simulink model "VehDymcModel_Outputer"  (R2022b)
settings: Solver=ode4  StartTime=0.0  StopTime=DrvCycLen  RelTol=1e-3
model workspace (MAT data in the model file):
  socvcb = containers.Map
  socvcb.serialization.keys = {}
  socvcb.serialization.values = {}
  socvcb.serialization.uniformity = 0
  socvcb.serialization.keyType = 'double'
  socvcb.serialization.valueType = 'any'
values from neighbouring files (symbols this model uses):
  DCAC_eff = 0.95    [FCEV_original_data.mat]
  m = Time_sample    [Config_c22100601.m]    (also in Config_c22100701.m)
  MC_eff_brk_average = 0.810578512397    [FCEV_original_data.mat]
  MC_eff_dri_average = 0.810578512397    [FCEV_original_data.mat]
  MC_inertia = 0.06    [FCEV_original_data.mat]
  MC_ori_eff = [0.7 0.78 0.85 0.86 0.81 0.82 0.79 0.78 0.78 0.78 0.78 0.7 ... (231 elements, 11x21)]    [FCEV_original_data.mat]
  MC_ori_power_brk_req_kW = [0 -28.3912930389 -56.7825860779 -85.1738791168 -113.565172156 -141.956465195 -170.347758234 -198.739051273 -227.130344311 -255.52163735 -283.912930389 0 ... (121 elements, 11x11)]    [FCEV_original_data.mat]
  MC_ori_power_dri_req_kW = [0 0 0 0 0 0 0 0 0 0 0 0 ... (121 elements, 11x11)]    [FCEV_original_data.mat]
  MC_ori_spd_rpm = [0 1000 2000 3000 4000 5000 6000 7000 8000 9000 10000]    [FCEV_original_data.mat]
  MC_ori_trq_brk_max_Nm = [-271.1368 -271.1368 -271.1368 -237.5159 -178.1369 -142.4824 -118.7579 -101.8119 -89.0685 -79.172 -71.1734]    [FCEV_original_data.mat]
  MC_ori_trq_brk_Nm = [-271.136848522 -244.02316367 -216.909478817 -189.795793965 -162.682109113 -135.568424261 -108.454739409 -81.3410545565 -54.2273697044 -27.1136848522 0]    [FCEV_original_data.mat]
  MC_ori_trq_dri_max_Nm = [271.1368 271.1368 271.1368 237.5159 178.1369 142.4824 118.7579 101.8119 89.0685 79.172 71.1734]    [FCEV_original_data.mat]
  MC_ori_trq_dri_Nm = [0 27.1136848522 54.2273697044 81.3410545565 108.454739409 135.568424261 162.682109113 189.795793965 216.909478817 244.02316367 271.136848522]    [FCEV_original_data.mat]
  MC_ori_trq_Nm = [-271.136848522 -244.02316367 -216.909478817 -189.795793965 -162.682109113 -135.568424261 -108.454739409 -81.3410545565 -54.2273697044 -27.1136848522 0 27.1136848522 ... (21 elements, 1x21)]    [FCEV_original_data.mat]
  MC_power_max_kW = 75    [FCEV_original_data.mat]
  MC_spd_max_rpm = 10000    [FCEV_original_data.mat]
  MC_spd_min_rpm = 0    [FCEV_original_data.mat]
  MC_spd_scale = 1    [FCEV_original_data.mat]
  MC_trq_scale = 1    [FCEV_original_data.mat]
  PredLen = 5    [Config_c221112.m]    (also in Config_c221127.m; Config_c221218.m; Config_c230117.m; Config_c230321.m)
  Road_u = 0.75    [FCEV_original_data.mat]
  SLMP_LearningRate = 0.05    [Config_c221112.m]    (also in Config_c221127.m; Config_c221218.m; Config_c230117.m; Config_c230321.m)
  Veh_air_density_kgpm2 = 1.2    [FCEV_original_data.mat]
  Veh_brk_front = [1 0.6 0.608 0.61 0.618 0.624 0.636 0.645 0.655]    [FCEV_original_data.mat]
  Veh_brk_z = [0.1 0.2 0.3 0.4 0.5 0.6 0.7 0.8 0.9]    [FCEV_original_data.mat]
  Veh_brk_z_max = 0.7    [FCEV_original_data.mat]
  Veh_brk_z_min = 0.1    [FCEV_original_data.mat]
  Veh_coeff_drag = 0.312    [FCEV_original_data.mat]
  Veh_coeff_roll = 0.00863    [FCEV_original_data.mat]
  Veh_final_drive_inertia = 0.1105    [FCEV_original_data.mat]
  Veh_final_drive_ratio = 3.47    [FCEV_original_data.mat]
  Veh_frontal_area_m2 = 2.06    [FCEV_original_data.mat]
  Veh_gravity_acc_ms2 = 9.81    [FCEV_original_data.mat]
  Veh_mass_cargo_kg = 113    [FCEV_original_data.mat]
  Veh_mass_curb_kg = 1157    [FCEV_original_data.mat]
  Veh_mech_eff = 0.9    [FCEV_original_data.mat]
  Veh_rotary_mass_conversion_factor = 1.05    [FCEV_original_data.mat]
  Veh_size_cg_height_m = 0.53    [FCEV_original_data.mat]
  Veh_wheel_inertia = 3.1039    [FCEV_original_data.mat]
  Veh_wheel_radius_m = 0.313    [FCEV_original_data.mat]
  Veh_wt_frac_front = 0.5    [FCEV_original_data.mat]
libraries: autolibshared x1
settings Model: Creator=xuupp  LastModifiedBy=xuupp
settings DataIOCC: ReturnWorkspaceOutputs=off

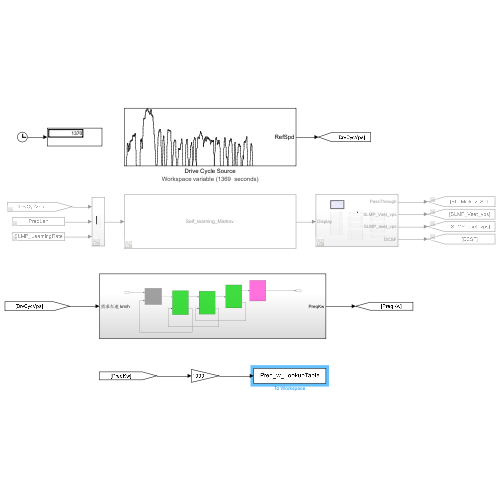
[thumbnail: Simulink's stored preview of the top-level diagram]
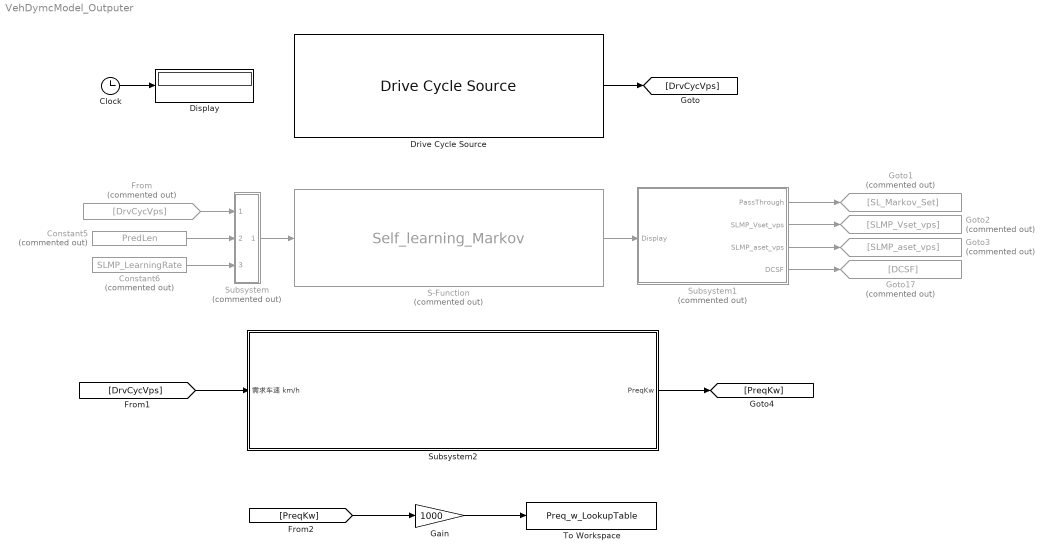
== system VehDymcModel_Outputer ==
  Clock : Clock
  Constant5 : Constant  Commented=on  Value=PredLen
  Constant6 : Constant  Commented=on  Value=SLMP_LearningRate
  Display : Display
  Drive Cycle Source : autolibshared/Drive Cycle Source  cycleVar=Workspace variable  wsVar=DrvCycVps  fileVar=cycleFTP75.mat  tfinal="1369  seconds"  cycleRepeat=off  outAccPort=off  outGearPort=off  gearList=No gear data  t_wot1=5  xdot_woto=0  xdot_wot1=30  t_wot2=20  xdot_wot2=0  t_wotend=30  srcUnit=m/s  outUnit=m/s  srcAccUnit=m/s/s  outAccUnit=m/s^2  dt=1  aMode=1  faultOption=off  velBnd=2  velBndUnit=mph  inUnit=m/s  timeBnd=1  failOption=off  stopSim=off  maxFaultCnt=10  maxFaultTime=2  maxTotFaultTime=15  traceOption=off  dtTrace=1  traceWindow=10  lastDCname=Custom Data Set  lastOutUnit=mph  lastDT=1  lastTB=1  lastSB=2  forceCalcBound=off
  From : From  Commented=on  GotoTag=DrvCycVps
  Gain : Gain  Gain=1000
  Goto1 : Goto  Commented=on  GotoTag=SL_Markov_Set
  Goto17 : Goto  Commented=on  GotoTag=DCSF
  Goto2 : Goto  Commented=on  GotoTag=SLMP_Vset_vps
  Goto3 : Goto  Commented=on  GotoTag=SLMP_aset_vps
  S-Function : S-Function  Commented=on  FunctionName=Self_learning_Markov  SFunctionDeploymentMode=off  EnableBusSupport=off
  Subsystem : Subsystem  Commented=on
  Subsystem1 : Subsystem  Commented=on
  Subsystem2 : Subsystem
  To Workspace : ToWorkspace  VariableName=Preq_w_LookupTable  SampleTime=-1
  wires:
  Subsystem1/1(PassThrough) -> Goto1/1
  S-Function/1 -> Subsystem1/1(Display)
  Subsystem1/2(SLMP_Vset_vps) -> Goto2/1
  Subsystem/1(HstLog) -> S-Function/1
  Subsystem1/3(SLMP_aset_vps) -> Goto3/1
  Constant5/1 -> Subsystem/2(RowSequence1)
  Clock/1 -> Display/1
  Subsystem1/4(DCSF) -> Goto17/1
  Constant6/1 -> Subsystem/3(RowSequence2)
  Drive Cycle Source/1 -> [DrvCycVps]
  From/1 -> Subsystem/1(RowSequence)
  [DrvCycVps] -> Subsystem2/1(需求车速 km/h)
  Subsystem2/1(PreqKw) -> [PreqKw]
  [PreqKw] -> Gain/1
  Gain/1 -> To Workspace/1

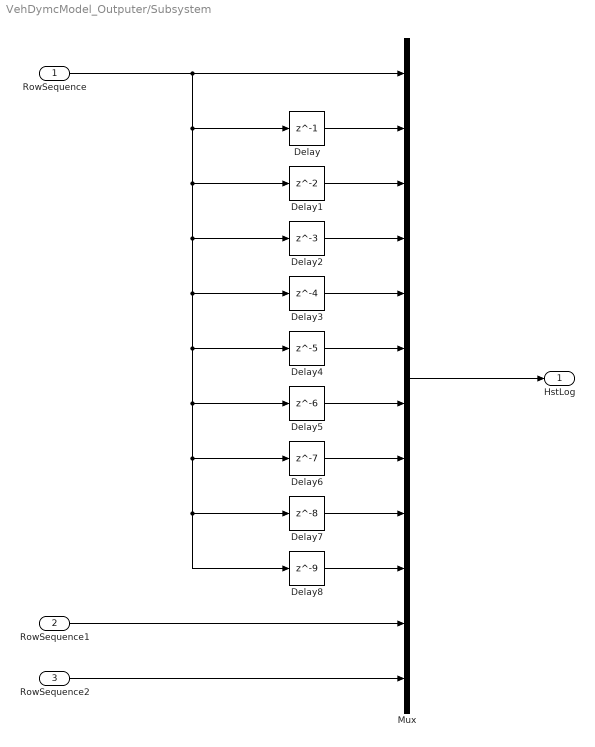
== system VehDymcModel_Outputer/Subsystem ==
  RowSequence : Inport
  RowSequence1 : Inport  Port=2
  RowSequence2 : Inport  Port=3
  Delay : Delay  DelayLength=1
  Delay1 : Delay
  Delay2 : Delay  DelayLength=3
  Delay3 : Delay  DelayLength=4
  Delay4 : Delay  DelayLength=5
  Delay5 : Delay  DelayLength=6
  Delay6 : Delay  DelayLength=7
  Delay7 : Delay  DelayLength=8
  Delay8 : Delay  DelayLength=9
  Mux : Mux  Inputs=12
  HstLog : Outport
  wires:
  RowSequence/1 -> Delay8/1, Delay7/1, Delay6/1, Delay5/1, Delay4/1, Delay3/1, Delay2/1, Delay1/1, Delay/1, Mux/1
  Mux/1 -> HstLog/1
  Delay8/1 -> Mux/10
  Delay7/1 -> Mux/9
  Delay6/1 -> Mux/8
  Delay5/1 -> Mux/7
  Delay3/1 -> Mux/5
  Delay2/1 -> Mux/4
  Delay1/1 -> Mux/3
  Delay/1 -> Mux/2
  Delay4/1 -> Mux/6
  RowSequence1/1 -> Mux/11
  RowSequence2/1 -> Mux/12

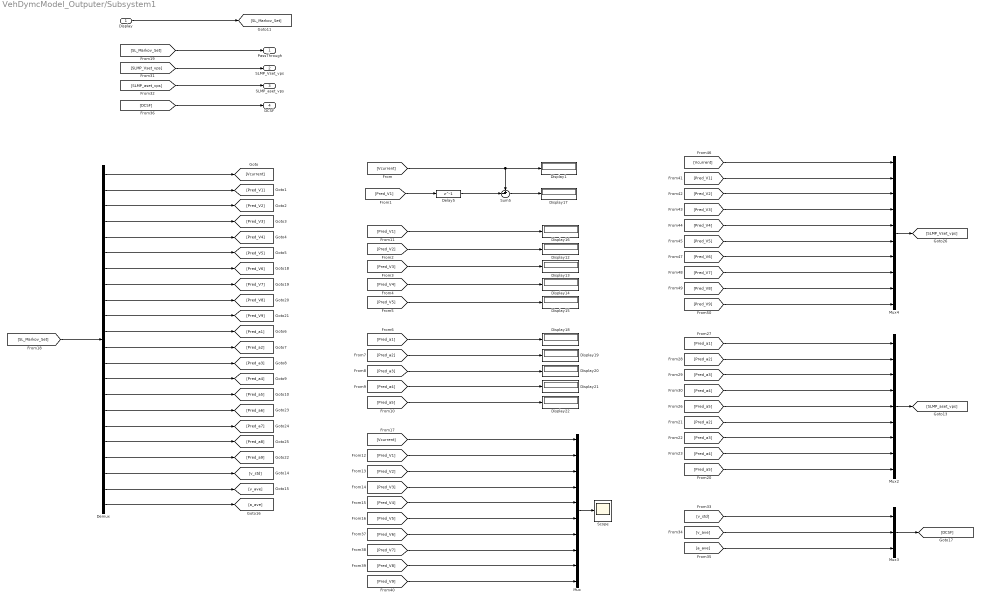
== system VehDymcModel_Outputer/Subsystem1 ==
  Display : Inport
  Delay5 : Delay  DelayLength=1
  Demux : Demux  Outputs=22
  Display{1,12..22} (12 alike) : Display
  Mux : Mux  Inputs=10
  Mux2 : Mux  Inputs=9
  Mux3 : Mux  Inputs=3
  Mux4 : Mux  Inputs=10
  Scope : Scope
  Sum5 : Sum  Inputs=+-|
  PassThrough : Outport
  SLMP_Vset_vps : Outport  Port=2
  SLMP_aset_vps : Outport  Port=3
  DCSF : Outport  Port=4
  wires:
  Display/1 -> [SL_Markov_Set]
  Demux/1 -> [Vcurrent]
  Demux/2 -> [Pred_V1]
  Demux/3 -> [Pred_V2]
  Demux/4 -> [Pred_V3]
  Demux/5 -> [Pred_V4]
  Demux/6 -> [Pred_V5]
  [Pred_V1] -> Delay5/1
  Delay5/1 -> Sum5/2
  [Pred_V2] -> Display12/1
  [Pred_V3] -> Display13/1
  [Vcurrent] -> Display1/1, Sum5/1
  Sum5/1 -> Display17/1
  [Pred_V4] -> Display14/1
  [Pred_V5] -> Display15/1
  [Pred_V1] -> Display16/1
  [Pred_a1] -> Display18/1
  [Pred_a2] -> Display19/1
  [Pred_a3] -> Display20/1
  [Pred_a4] -> Display21/1
  [Pred_a5] -> Display22/1
  Mux/1 -> Scope/1
  [Pred_V5] -> Mux/6
  [Pred_V4] -> Mux/5
  [Pred_V3] -> Mux/4
  [Pred_V2] -> Mux/3
  [Pred_V1] -> Mux/2
  [Vcurrent] -> Mux/1
  [SL_Markov_Set] -> Demux/1
  [SL_Markov_Set] -> PassThrough/1
  [Pred_a3] -> Mux2/3
  [Pred_a2] -> Mux2/2
  [Pred_a1] -> Mux2/1
  [Pred_a4] -> Mux2/4
  [Pred_a5] -> Mux2/5
  Mux2/1 -> [SLMP_aset_vps]
  [SLMP_Vset_vps] -> SLMP_Vset_vps/1
  [SLMP_aset_vps] -> SLMP_aset_vps/1
  [v_std] -> Mux3/1
  [v_ave] -> Mux3/2
  [a_ave] -> Mux3/3
  Mux3/1 -> [DCSF]
  [DCSF] -> DCSF/1
  Demux/7 -> [Pred_V6]
  Demux/8 -> [Pred_V7]
  Demux/9 -> [Pred_V8]
  Demux/10 -> [Pred_V9]
  Demux/11 -> [Pred_a1]
  Demux/12 -> [Pred_a2]
  Demux/13 -> [Pred_a3]
  Demux/14 -> [Pred_a4]
  Demux/15 -> [Pred_a5]
  Demux/16 -> [Pred_a6]
  Demux/17 -> [Pred_a7]
  Demux/18 -> [Pred_a8]
  Demux/19 -> [Pred_a9]
  Demux/20 -> [v_std]
  Demux/21 -> [v_ave]
  Demux/22 -> [a_ave]
  [Pred_V6] -> Mux/7
  [Pred_V9] -> Mux/10
  [Pred_V7] -> Mux/8
  [Pred_V8] -> Mux/9
  [Pred_V8] -> Mux4/9
  [Pred_V7] -> Mux4/8
  [Pred_V9] -> Mux4/10
  [Pred_V6] -> Mux4/7
  [Vcurrent] -> Mux4/1
  [Pred_V1] -> Mux4/2
  [Pred_V2] -> Mux4/3
  [Pred_V3] -> Mux4/4
  [Pred_V4] -> Mux4/5
  [Pred_V5] -> Mux4/6
  Mux4/1 -> [SLMP_Vset_vps]
  [Pred_a2] -> Mux2/6
  [Pred_a3] -> Mux2/7
  [Pred_a4] -> Mux2/8
  [Pred_a5] -> Mux2/9

== system VehDymcModel_Outputer/Subsystem2 ==
  需求车速 km/h : Inport
  Power bus : Subsystem
  主减及变速器模型 : Subsystem
  整车动力学模型 : Subsystem
  车轮模型 : Subsystem
  驱动电机模型 : Subsystem
  PreqKw : Outport
  wires:
  驱动电机模型/2(drive torque (Nm) brake torque (Nm) speed avail (rad/s) avail. at rotor) -> 主减及变速器模型/2(drive torque (Nm) brake torque (Nm) speed avail (rad/s) at input side of final drive)
  车轮模型/1(drive torque (Nm) speed (rad/s) brake torque (Nm) req'd from drivetrain into axle) -> 主减及变速器模型/1(drive torque (Nm) speed (rad/s) brake torque (Nm) req'd at output side of final drive)
  整车动力学模型/1(需求驱动力N 目标车速m/s 需求制动力N) -> 车轮模型/1("tractive force, brake force and speed req'd of tire/road interface 需求驱动力N 目标车速m/s 需求制动力N")
  主减及变速器模型/2(drive torque (Nm) brake torque (Nm) speed avail (rad/s) at output side of final drive) -> 车轮模型/2("drive torque (Nm) brake torque (Nm) speed (rad/s) available from drivetrain into axle ")
  主减及变速器模型/1(drive torque (Nm) speed (rad/s) brike torque (Nm) req'd at input side of final drive) -> 驱动电机模型/1(drive torque (Nm) speed (rad/s) brake torque (Nm) req'd at motor)
  驱动电机模型/1(drive power (kW) brake power (kW) req'd motor input power (电功率)) -> Power bus/1(drive power (kW) brake power (kW) req at power bus)
  车轮模型/2(tractive force (N) brake force (N) linear speed achievable (m/s)) -> 整车动力学模型/2(实际车辆驱动力N 制动力N 和车速m/s)
  Power bus/1(PreqKw) -> PreqKw/1
  需求车速 km/h/1 -> 整车动力学模型/1(需求车速 km/h)

== system VehDymcModel_Outputer/Subsystem2/Power bus ==
  note: -
  note: +
  note: 需求制动功率
  note: 需求驱动功率
  drive power (kW) brake power (kW) req at power bus : Inport
  Constant1 : Constant  Value=DCAC_eff
  Demux2 : Demux  Outputs=2
  Divide : Product  Inputs=*/
  Divide1 : Product  Inputs=**
  Saturation : Saturate  UpperLimit=0  LowerLimit=-inf
  Saturation1 : Saturate  UpperLimit=inf  LowerLimit=0
  Switch1 : Switch  Criteria=u2 > Threshold  SaturateOnIntegerOverflow=off  InputSameDT=off
  PreqKw : Outport
  wires:
  Constant1/1 -> Divide1/2, Divide/2
  Divide/1 -> Saturation1/1
  Divide1/1 -> Saturation/1
  drive power (kW) brake power (kW) req at power bus/1 -> Demux2/1
  Demux2/2 -> Divide1/1
  Saturation1/1 -> Switch1/2, Switch1/1
  Switch1/1 -> PreqKw/1
  Saturation/1 -> Switch1/3
  Demux2/1 -> Divide/1

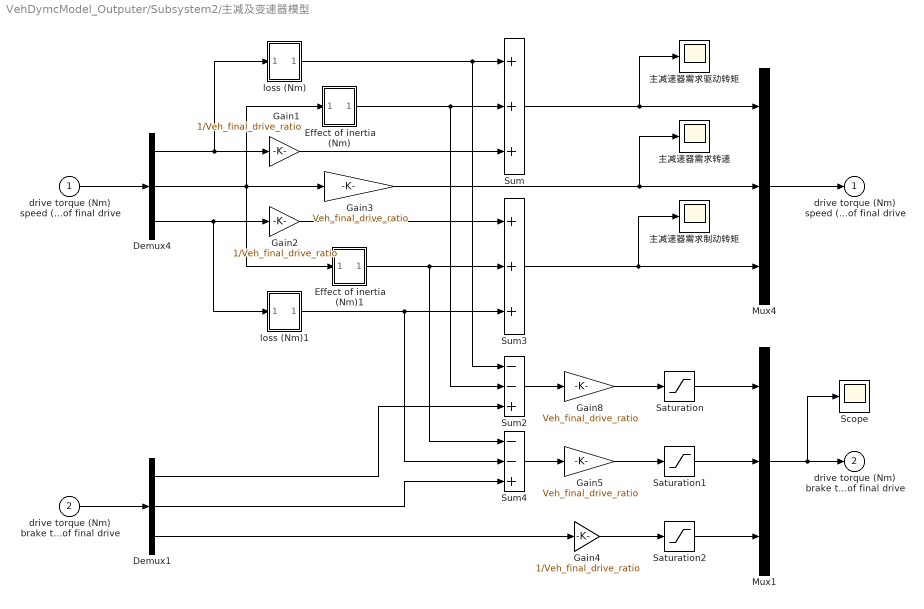
== system VehDymcModel_Outputer/Subsystem2/主减及变速器模型 ==
  drive torque (Nm) speed (rad/s) brake torque (Nm) req'd at output side of final drive : Inport
  drive torque (Nm) brake torque (Nm) speed avail (rad/s) at input side of final drive : Inport  Port=2
  " Effect of inertia (Nm)1" : Subsystem
  Demux1 : Demux  Outputs=3
  Demux4 : Demux  Outputs=3
  Effect of inertia (Nm) : Subsystem
  Gain1 : Gain  Gain=1/Veh_final_drive_ratio
  Gain2 : Gain  Gain=1/Veh_final_drive_ratio
  Gain3 : Gain  Gain=Veh_final_drive_ratio  SaturateOnIntegerOverflow=on  OutDataTypeStr=Inherit: Same as input  ParamDataTypeStr=Inherit: Same as input
  Gain4 : Gain  Gain=1/Veh_final_drive_ratio  SaturateOnIntegerOverflow=on  OutDataTypeStr=Inherit: Same as input  ParamDataTypeStr=Inherit: Same as input
  Gain5 : Gain  Gain=Veh_final_drive_ratio  SaturateOnIntegerOverflow=on  OutDataTypeStr=Inherit: Same as input  ParamDataTypeStr=Inherit: Same as input
  Gain8 : Gain  Gain=Veh_final_drive_ratio  SaturateOnIntegerOverflow=on  OutDataTypeStr=Inherit: Same as input  ParamDataTypeStr=Inherit: Same as input
  Mux1 : Mux  Inputs=3
  Mux4 : Mux  Inputs=3
  Saturation : Saturate  UpperLimit=inf  LowerLimit=0
  Saturation1 : Saturate  UpperLimit=0  LowerLimit=-inf
  Saturation2 : Saturate  UpperLimit=inf  LowerLimit=0
  Scope : Scope
  Sum : Sum  Inputs=+++  InputSameDT=on  SaturateOnIntegerOverflow=on  OutDataTypeStr=Inherit: Same as first input
  Sum2 : Sum  Inputs=--+  InputSameDT=on  SaturateOnIntegerOverflow=on  OutDataTypeStr=Inherit: Same as first input
  Sum3 : Sum  Inputs=+++  InputSameDT=on  SaturateOnIntegerOverflow=on  OutDataTypeStr=Inherit: Same as first input
  Sum4 : Sum  Inputs=--+  InputSameDT=on  SaturateOnIntegerOverflow=on  OutDataTypeStr=Inherit: Same as first input
  loss (Nm) : Subsystem
  loss (Nm)1 : Subsystem
  主减速器需求制动转矩 : Scope
  主减速器需求转速 : Scope
  主减速器需求驱动转矩 : Scope
  drive torque (Nm) speed (rad/s) brike torque (Nm) req'd at input side of final drive : Outport  InitialOutput=0
  drive torque (Nm) brake torque (Nm) speed avail (rad/s) at output side of final drive : Outport  Port=2  InitialOutput=0
  wires:
  Demux4/2 -> Effect of inertia (Nm)/1(fd input speed (rad/s)), " Effect of inertia (Nm)1"/1(In1), Gain3/1
  Demux4/1 -> loss (Nm)/1("drive torque (Nm) "), Gain1/1
  Mux4/1 -> drive torque (Nm) speed (rad/s) brike torque (Nm) req'd at input side of final drive/1
  drive torque (Nm) speed (rad/s) brake torque (Nm) req'd at output side of final drive/1 -> Demux4/1
  Mux1/1 -> Scope/1, drive torque (Nm) brake torque (Nm) speed avail (rad/s) at output side of final drive/1
  drive torque (Nm) brake torque (Nm) speed avail (rad/s) at input side of final drive/1 -> Demux1/1
  Effect of inertia (Nm)/1(drag torque (Nm)) -> Sum2/2, Sum/2
  loss (Nm)/1(drag torque (Nm)) -> Sum2/1, Sum/1
  Gain1/1 -> Sum/3
  Sum/1 -> 主减速器需求驱动转矩/1, Mux4/1
  Gain3/1 -> 主减速器需求转速/1, Mux4/2
  " Effect of inertia (Nm)1"/1(Out1) -> Sum4/1, Sum3/2
  loss (Nm)1/1(drag torque (Nm)) -> Sum4/2, Sum3/3
  Demux4/3 -> Gain2/1, loss (Nm)1/1("drive torque (Nm) ")
  Gain2/1 -> Sum3/1
  Demux1/1 -> Sum2/3
  Demux1/2 -> Sum4/3
  Sum2/1 -> Gain8/1
  Gain8/1 -> Saturation/1
  Saturation/1 -> Mux1/1
  Sum4/1 -> Gain5/1
  Saturation1/1 -> Mux1/2
  Gain5/1 -> Saturation1/1
  Gain4/1 -> Saturation2/1
  Demux1/3 -> Gain4/1
  Saturation2/1 -> Mux1/3
  Sum3/1 -> 主减速器需求制动转矩/1, Mux4/3

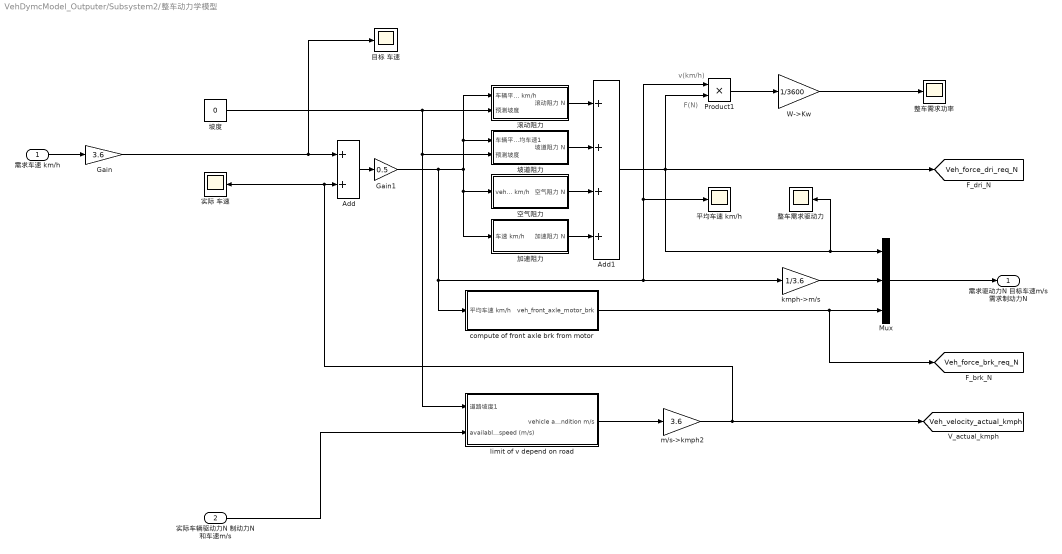
== system VehDymcModel_Outputer/Subsystem2/整车动力学模型 ==
  note: v(km/h)
  note: F(N)
  需求车速 km/h : Inport
  实际车辆驱动力N 制动力N 和车速m/s : Inport  Port=2
  Add : Sum
  Add1 : Sum  Inputs=++++
  Gain : Gain  Gain=3.6
  Gain1 : Gain  Gain=0.5
  Mux : Mux  Inputs=3
  Product1 : Product  RndMeth=Zero
  W->Kw : Gain  Gain=1/3600
  compute of front axle brk from motor : Subsystem
  kmph->m/s : Gain  Gain=1/3.6
  limit of v depend on road : Subsystem
  m/s->kmph2 : Gain  Gain=3.6
  加速阻力 : Subsystem
  坡度 : Constant  Value=0
  坡道阻力 : Subsystem
  实际 车速 : Scope
  平均车速 km/h : Scope
  整车需求功率 : Scope
  整车需求驱动力 : Scope
  滚动阻力 : Subsystem
  目标 车速 : Scope
  空气阻力 : Subsystem
  需求驱动力N 目标车速m/s 需求制动力N : Outport
  tag scope: Veh_force_brk_req_N=global, Veh_force_dri_req_N=global, Veh_velocity_actual_kmph=global
  wires:
  需求车速 km/h/1 -> Gain/1
  Add/1 -> Gain1/1
  实际车辆驱动力N 制动力N 和车速m/s/1 -> limit of v depend on road/2(available drive force (N) brake force (N) and linear speed (m/s))
  滚动阻力/1(滚动阻力 N) -> Add1/1
  坡道阻力/1(坡道阻力 N) -> Add1/2
  空气阻力/1(空气阻力 N) -> Add1/3
  加速阻力/1(加速阻力 N) -> Add1/4
  Add1/1 -> 整车需求驱动力/1, Mux/1, [Veh_force_dri_req_N], Product1/2
  Mux/1 -> 需求驱动力N 目标车速m/s 需求制动力N/1
  Product1/1 -> W->Kw/1
  坡度/1 -> limit of v depend on road/1(道路坡度1), 坡道阻力/2(预测坡度), 滚动阻力/2(预测坡度)
  W->Kw/1 -> 整车需求功率/1
  kmph->m/s/1 -> Mux/2
  limit of v depend on road/1(vehicle achievable consider of the road condition m/s) -> m/s->kmph2/1
  m/s->kmph2/1 -> 实际 车速/1, Add/2, [Veh_velocity_actual_kmph]
  Gain1/1 -> compute of front axle brk from motor/1(平均车速 km/h), kmph->m/s/1, 平均车速 km/h/1, Product1/1, 加速阻力/1(车速 km/h), 空气阻力/1(veh_spd km/h), 滚动阻力/1(车辆平均车速 km/h), 坡道阻力/1(车辆平均车速1)
  compute of front axle brk from motor/1(veh_front_axle_motor_brk) -> Mux/3, [Veh_force_brk_req_N]
  Gain/1 -> Add/1, 目标 车速/1

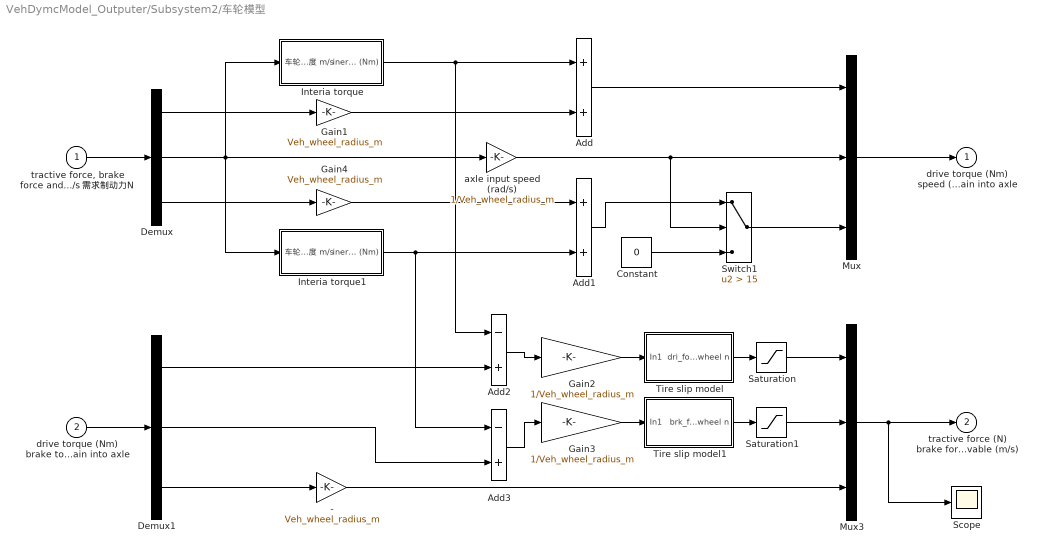
== system VehDymcModel_Outputer/Subsystem2/车轮模型 ==
  "tractive force, brake force and speed req'd of tire/road interface 需求驱动力N 目标车速m/s 需求制动力N" : Inport
  "drive torque (Nm) brake torque (Nm) speed (rad/s) available from drivetrain into axle " : Inport  Port=2
  - : Gain  Gain=Veh_wheel_radius_m
  Add : Sum
  Add1 : Sum
  Add2 : Sum  Inputs=-+
  Add3 : Sum  Inputs=-+
  Constant : Constant  Value=0
  Demux : Demux  Outputs=3
  Demux1 : Demux  Outputs=3
  Gain1 : Gain  Gain=Veh_wheel_radius_m
  Gain2 : Gain  Gain=1/Veh_wheel_radius_m
  Gain3 : Gain  Gain=1/Veh_wheel_radius_m
  Gain4 : Gain  Gain=Veh_wheel_radius_m
  Interia torque : Subsystem
  Interia torque1 : Subsystem
  Mux : Mux  Inputs=3
  Mux3 : Mux  Inputs=3
  Saturation : Saturate  UpperLimit=inf  LowerLimit=0
  Saturation1 : Saturate  UpperLimit=0  LowerLimit=-inf
  Scope : Scope
  Switch1 : Switch  Criteria=u2 > Threshold  Threshold=15  SaturateOnIntegerOverflow=off  InputSameDT=off
  Tire slip model : Subsystem
  Tire slip model1 : Subsystem
  axle input speed (rad/s) : Gain  Gain=1/Veh_wheel_radius_m
  drive torque (Nm) speed (rad/s) brake torque (Nm) req'd from drivetrain into axle : Outport  InitialOutput=0
  tractive force (N) brake force (N) linear speed achievable (m/s) : Outport  Port=2  InitialOutput=0
  wires:
  Demux/1 -> Gain1/1
  "tractive force, brake force and speed req'd of tire/road interface 需求驱动力N 目标车速m/s 需求制动力N"/1 -> Demux/1
  "drive torque (Nm) brake torque (Nm) speed (rad/s) available from drivetrain into axle "/1 -> Demux1/1
  Demux1/1 -> Add2/2
  Mux/1 -> drive torque (Nm) speed (rad/s) brake torque (Nm) req'd from drivetrain into axle/1
  Gain1/1 -> Add/2
  Add/1 -> Mux/1
  Add2/1 -> Gain2/1
  Gain2/1 -> Tire slip model/1(In1)
  Mux3/1 -> Scope/1, tractive force (N) brake force (N) linear speed achievable (m/s)/1
  Demux/2 -> axle input speed (rad/s)/1, Interia torque/1(车轮线速度 m/s), Interia torque1/1(车轮线速度 m/s)
  Interia torque/1(inertia torque (Nm)) -> Add2/1, Add/1
  Demux/3 -> Gain4/1
  Gain4/1 -> Add1/1
  Interia torque1/1(inertia torque (Nm)) -> Add3/1, Add1/2
  axle input speed (rad/s)/1 -> Switch1/2, Mux/2
  Switch1/1 -> Mux/3
  Constant/1 -> Switch1/3
  Add1/1 -> Switch1/1
  Saturation/1 -> Mux3/1
  Tire slip model/1(dri_force available in front wheel n) -> Saturation/1
  Tire slip model1/1(brk_force available in front wheel n) -> Saturation1/1
  Saturation1/1 -> Mux3/2
  Gain3/1 -> Tire slip model1/1(In1)
  Demux1/2 -> Add3/2
  Add3/1 -> Gain3/1
  Demux1/3 -> -/1
  -/1 -> Mux3/3

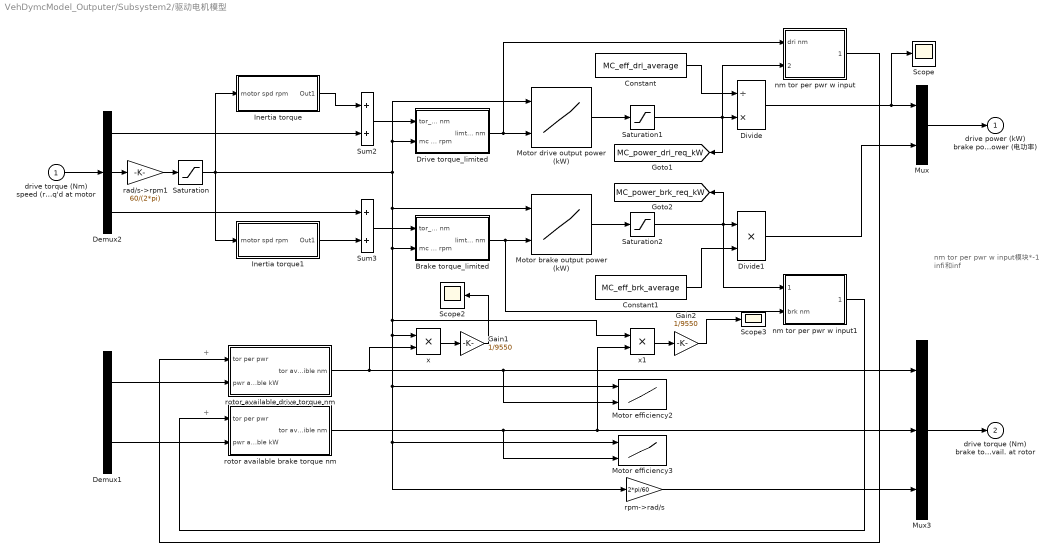
== system VehDymcModel_Outputer/Subsystem2/驱动电机模型 ==
  note: +
  note: +
  note: nm tor per pwr w input模块*-1
      | infi和inf
  drive torque (Nm) speed (rad/s) brake torque (Nm) req'd at motor : Inport
  Brake torque_limited : Subsystem
  Constant : Constant  Value=MC_eff_dri_average
  Constant1 : Constant  Value=MC_eff_brk_average
  Demux1 : Demux  Outputs=2
  Demux2 : Demux  Outputs=3
  Divide : Product  Inputs=/*
  Divide1 : Product  Inputs=**
  Drive torque_limited : Subsystem
  Gain1 : Gain  Gain=1/9550
  Gain2 : Gain  Gain=1/9550
  Inertia torque : Subsystem
  Inertia torque1 : Subsystem
  Motor brake output power (kW) : Lookup2D  RowIndex=MC_ori_spd_rpm*MC_spd_scale  ColumnIndex=MC_ori_trq_brk_Nm*MC_trq_scale  Table=MC_ori_power_brk_req_kW*MC_spd_scale*MC_trq_scale
  Motor drive output power (kW) : Lookup2D  RowIndex=MC_ori_spd_rpm*MC_spd_scale  ColumnIndex=MC_ori_trq_dri_Nm*MC_trq_scale  Table=MC_ori_power_dri_req_kW*MC_spd_scale*MC_trq_scale
  Motor efficiency2 : Lookup2D  RowIndex=MC_ori_spd_rpm*MC_spd_scale  ColumnIndex=MC_ori_trq_Nm*MC_trq_scale  Table=MC_ori_eff*MC_spd_scale*MC_trq_scale
  Motor efficiency3 : Lookup2D  RowIndex=MC_ori_spd_rpm*MC_spd_scale  ColumnIndex=MC_ori_trq_Nm*MC_trq_scale  Table=MC_ori_eff*MC_spd_scale*MC_trq_scale
  Mux : Mux  Inputs=2
  Mux3 : Mux  Inputs=3
  Saturation : Saturate  UpperLimit=MC_spd_max_rpm  LowerLimit=MC_spd_min_rpm
  Saturation1 : Saturate  UpperLimit=MC_power_max_kW  LowerLimit=0  LinearizeAsGain=off
  Saturation2 : Saturate  UpperLimit=0  LowerLimit=-MC_power_max_kW
  Scope : Scope
  Scope2 : Scope
  Scope3 : Scope
  Sum2 : Sum  InputSameDT=on  SaturateOnIntegerOverflow=on  OutDataTypeStr=Inherit: Same as first input
  Sum3 : Sum  InputSameDT=on  SaturateOnIntegerOverflow=on  OutDataTypeStr=Inherit: Same as first input
  nm tor per pwr w input : Subsystem
  nm tor per pwr w input1 : Subsystem
  rad/s->rpm1 : Gain  Gain=60/(2*pi)
  rotor available brake torque nm : Subsystem
  rotor available drive torque nm : Subsystem
  rpm->rad/s : Gain  Gain=2*pi/60
  x : Product  Inputs=**
  x1 : Product  Inputs=**
  drive power (kW) brake power (kW) req'd motor input power (电功率) : Outport  InitialOutput=0
  drive torque (Nm) brake torque (Nm) speed avail (rad/s) avail. at rotor : Outport  Port=2  InitialOutput=0
  tag scope: MC_power_brk_req_kW=global, MC_power_dri_req_kW=global
  wires:
  drive torque (Nm) speed (rad/s) brake torque (Nm) req'd at motor/1 -> Demux2/1
  rad/s->rpm1/1 -> Saturation/1
  Demux2/2 -> rad/s->rpm1/1
  Demux2/1 -> Sum2/2
  Inertia torque/1(Out1) -> Sum2/1
  Sum2/1 -> Drive torque_limited/1(tor_req nm)
  Drive torque_limited/1(limted mc torque nm) -> Motor drive output power (kW)/2, nm tor per pwr w input/1(dri nm)
  Motor drive output power (kW)/1 -> Saturation1/1
  Constant/1 -> Divide/1
  Divide/1 -> Scope/1, Mux/1
  Mux/1 -> drive power (kW) brake power (kW) req'd motor input power (电功率)/1
  Demux2/3 -> Sum3/1
  Inertia torque1/1(Out1) -> Sum3/2
  Sum3/1 -> Brake torque_limited/1(tor_req nm)
  Motor brake output power (kW)/1 -> Saturation2/1
  Saturation2/1 -> [MC_power_brk_req_kW], nm tor per pwr w input1/1(pwr brk kW), Divide1/1
  Constant1/1 -> Divide1/2
  Divide1/1 -> Mux/2
  Saturation1/1 -> nm tor per pwr w input/2(pwr dri kW), [MC_power_dri_req_kW], Divide/2
  Demux1/1 -> rotor available drive torque nm/2(pwr available kW)
  nm tor per pwr w input/1(tor per pwr) -> rotor available drive torque nm/1(tor per pwr)
  Demux1/2 -> rotor available brake torque nm/2(pwr available kW)
  nm tor per pwr w input1/1(tor per pwr) -> rotor available brake torque nm/1(tor per pwr)
  rotor available brake torque nm/1(tor avaible nm) -> Motor efficiency3/2, x1/2, Mux3/2
  rotor available drive torque nm/1(tor avaible nm) -> Motor efficiency2/2, Mux3/1, x/2
  rpm->rad/s/1 -> Mux3/3
  Brake torque_limited/1(limted mc torque nm) -> nm tor per pwr w input1/2(brk nm), Motor brake output power (kW)/2
  Gain1/1 -> Scope2/1
  x/1 -> Gain1/1
  Gain2/1 -> Scope3/1
  x1/1 -> Gain2/1
  Saturation/1 -> Inertia torque1/1(motor spd rpm), x1/1, x/1, Motor efficiency2/1, Motor efficiency3/1, rpm->rad/s/1, Brake torque_limited/2(mc spd rpm), Motor brake output power (kW)/1, Motor drive output power (kW)/1, Drive torque_limited/2(mc spd rpm), Inertia torque/1(motor spd rpm)
  Mux3/1 -> drive torque (Nm) brake torque (Nm) speed avail (rad/s) avail. at rotor/1

== system VehDymcModel_Outputer/Subsystem2/主减及变速器模型/ Effect of inertia (Nm)1 ==
  In1 : Inport
  Constant : Constant  Value=0
  Derivative : Derivative
  Switch : Switch  SaturateOnIntegerOverflow=off  InputSameDT=off
  inertia : Gain  Gain=Veh_final_drive_inertia
  Out1 : Outport
  wires:
  inertia/1 -> Out1/1
  In1/1 -> Derivative/1
  Derivative/1 -> Switch/3, Switch/2
  Constant/1 -> Switch/1
  Switch/1 -> inertia/1

== system VehDymcModel_Outputer/Subsystem2/主减及变速器模型/Effect of inertia (Nm) ==
  note: The inertia torque is the input torque required to accelerate the
      | final drive's inertia as measured on the input side.
  fd input speed (rad/s) : Inport
  Gain : Gain  Gain=Veh_final_drive_inertia  SaturateOnIntegerOverflow=on  OutDataTypeStr=Inherit: Same as input  ParamDataTypeStr=Inherit: Same as input
  d/dt : Derivative
  drag torque (Nm) : Outport  InitialOutput=0
  wires:
  fd input speed (rad/s)/1 -> d/dt/1
  d/dt/1 -> Gain/1
  Gain/1 -> drag torque (Nm)/1

== system VehDymcModel_Outputer/Subsystem2/主减及变速器模型/loss (Nm) ==
  note: The loss torque is zero when the gears are not turning,
      | and is applied at the input side of the gear reduction.
  "drive torque (Nm) " : Inport
  Add : Sum  Inputs=+-
  Gain : Gain  Gain=1/Veh_mech_eff
  Gain1 : Gain  Gain=1/Veh_final_drive_ratio
  drag torque (Nm) : Outport  InitialOutput=0
  wires:
  Add/1 -> drag torque (Nm)/1
  "drive torque (Nm) "/1 -> Gain1/1
  Gain1/1 -> Add/2, Gain/1
  Gain/1 -> Add/1

== system VehDymcModel_Outputer/Subsystem2/主减及变速器模型/loss (Nm)1 ==
  note: The loss torque is zero when the gears are not turning,
      | and is applied at the input side of the gear reduction.
  "drive torque (Nm) " : Inport
  Add : Sum  Inputs=+-
  Gain : Gain  Gain=1/Veh_mech_eff
  Gain1 : Gain  Gain=1/Veh_final_drive_ratio
  drag torque (Nm) : Outport  InitialOutput=0
  wires:
  Add/1 -> drag torque (Nm)/1
  "drive torque (Nm) "/1 -> Gain1/1
  Gain1/1 -> Add/2, Gain/1
  Gain/1 -> Add/1

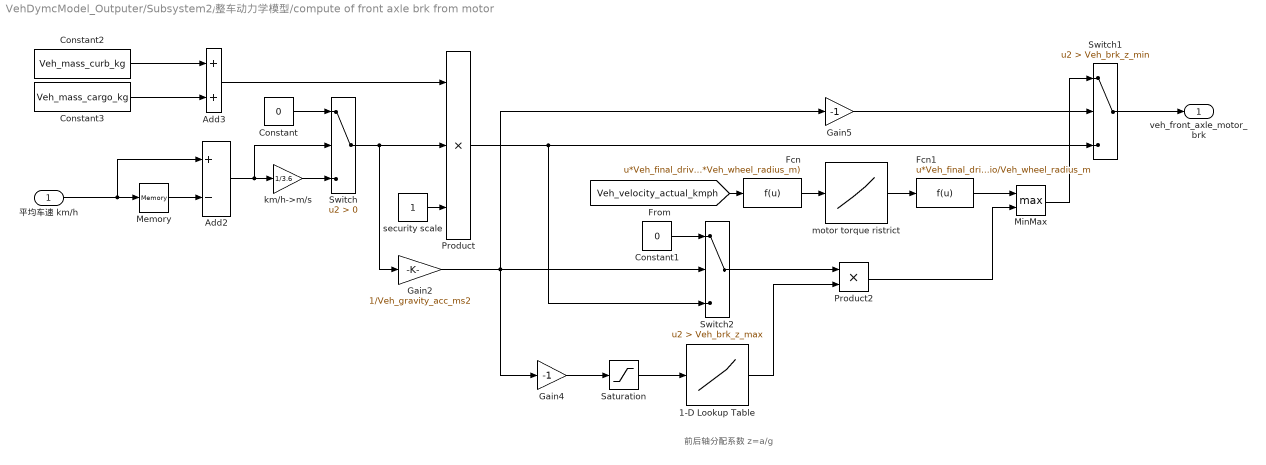
== system VehDymcModel_Outputer/Subsystem2/整车动力学模型/compute of front axle brk from motor ==
  note: 前后轴分配系数
      | z=a/g
  平均车速 km/h : Inport
  " security scale" : Constant
  1-D Lookup Table : Lookup_n-D  NumberOfTableDimensions=1  BreakpointsForDimension1=Veh_brk_z  Table=Veh_brk_front  RndMeth=Simplest
  Add2 : Sum  Inputs=+-
  Add3 : Sum
  Constant : Constant  Value=0
  Constant1 : Constant  Value=0
  Constant2 : Constant  Value=Veh_mass_curb_kg
  Constant3 : Constant  Value=Veh_mass_cargo_kg
  Fcn : Fcn  Expr=u*Veh_final_drive_ratio/(0.377*Veh_wheel_radius_m)
  Fcn1 : Fcn  Expr=u*Veh_final_drive_ratio/Veh_wheel_radius_m
  Gain2 : Gain  Gain=1/Veh_gravity_acc_ms2
  Gain4 : Gain  Gain=-1
  Gain5 : Gain  Gain=-1
  Memory : Memory  InheritSampleTime=on
  MinMax : MinMax  Function=max  Inputs=2
  Product : Product  Inputs=3  RndMeth=Zero
  Product2 : Product  RndMeth=Zero
  Saturation : Saturate  UpperLimit=Veh_brk_z_max  LowerLimit=Veh_brk_z_min
  Switch : Switch  Criteria=u2 > Threshold  SaturateOnIntegerOverflow=off  InputSameDT=off
  Switch1 : Switch  Criteria=u2 > Threshold  Threshold=Veh_brk_z_min  SaturateOnIntegerOverflow=off  InputSameDT=off
  Switch2 : Switch  Criteria=u2 > Threshold  Threshold=Veh_brk_z_max  SaturateOnIntegerOverflow=off  InputSameDT=off
  km/h->m/s : Gain  Gain=1/3.6
  motor torque ristrict : Lookup_n-D  NumberOfTableDimensions=1  BreakpointsForDimension1=MC_ori_spd_rpm  Table=MC_ori_trq_brk_max_Nm  RndMeth=Simplest
  veh_front_axle_motor_brk : Outport
  wires:
  Memory/1 -> Add2/2
  Add2/1 -> Switch/2, km/h->m/s/1
  km/h->m/s/1 -> Switch/3
  Constant/1 -> Switch/1
  Switch/1 -> Product/2, Gain2/1
  " security scale"/1 -> Product/3
  Gain2/1 -> Gain4/1, Gain5/1, Switch2/2
  Constant2/1 -> Add3/1
  Constant3/1 -> Add3/2
  Add3/1 -> Product/1
  Product/1 -> Switch1/3, Switch2/3
  Constant1/1 -> Switch2/1
  Gain4/1 -> Saturation/1
  Saturation/1 -> 1-D Lookup Table/1
  Switch2/1 -> Product2/1
  1-D Lookup Table/1 -> Product2/2
  Fcn/1 -> motor torque ristrict/1
  [Veh_velocity_actual_kmph] -> Fcn/1
  motor torque ristrict/1 -> Fcn1/1
  Fcn1/1 -> MinMax/1
  Product2/1 -> MinMax/2
  MinMax/1 -> Switch1/1
  Switch1/1 -> veh_front_axle_motor_brk/1
  Gain5/1 -> Switch1/2
  平均车速 km/h/1 -> Add2/1, Memory/1

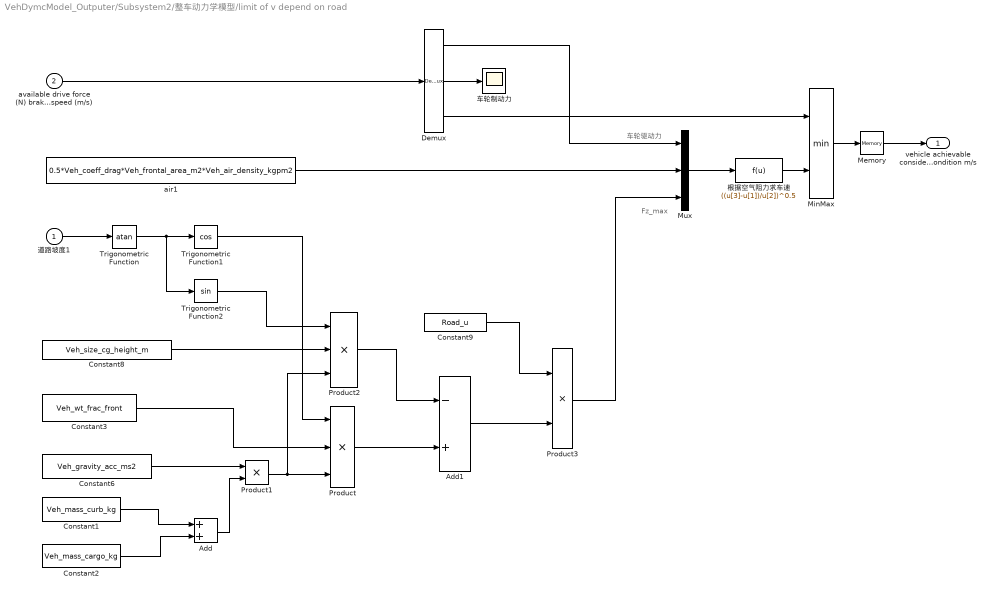
== system VehDymcModel_Outputer/Subsystem2/整车动力学模型/limit of v depend on road ==
  note: Fz_max
  note: 车轮驱动力
  道路坡度1 : Inport
  available drive force (N) brake force (N) and linear speed (m/s) : Inport  Port=2
  Add : Sum
  Add1 : Sum  Inputs=-+
  Constant1 : Constant  Value=Veh_mass_curb_kg
  Constant2 : Constant  Value=Veh_mass_cargo_kg
  Constant3 : Constant  Value=Veh_wt_frac_front
  Constant6 : Constant  Value=Veh_gravity_acc_ms2
  Constant8 : Constant  Value=Veh_size_cg_height_m
  Constant9 : Constant  Value=Road_u
  Demux : Demux  Outputs=3
      settings: DisplayOption=none
  Memory : Memory  InheritSampleTime=on
  MinMax : MinMax  Inputs=2
  Mux : Mux  Inputs=3
  Product : Product  Inputs=3  RndMeth=Zero
  Product1 : Product  RndMeth=Zero
  Product2 : Product  Inputs=3  RndMeth=Zero
  Product3 : Product  RndMeth=Zero
  Trigonometric Function : Trigonometry  Operator=atan
  Trigonometric Function1 : Trigonometry  Operator=cos
  Trigonometric Function2 : Trigonometry
  air1 : Constant  Value=0.5*Veh_coeff_drag*Veh_frontal_area_m2*Veh_air_density_kgpm2
  根据空气阻力求车速 : Fcn  Expr=((u[3]-u[1])/u[2])^0.5
  车轮制动力 : Scope
  vehicle achievable consider of the road condition m/s : Outport
  wires:
  air1/1 -> Mux/2
  Product3/1 -> Mux/3
  Mux/1 -> 根据空气阻力求车速/1
  Constant1/1 -> Add/1
  Constant2/1 -> Add/2
  道路坡度1/1 -> Trigonometric Function/1
  Trigonometric Function/1 -> Trigonometric Function2/1, Trigonometric Function1/1
  Trigonometric Function1/1 -> Product/1
  Add/1 -> Product1/2
  Constant6/1 -> Product1/1
  Product1/1 -> Product/3, Product2/3
  Constant3/1 -> Product/2
  Trigonometric Function2/1 -> Product2/1
  Constant8/1 -> Product2/2
  Product2/1 -> Add1/1
  Product/1 -> Add1/2
  根据空气阻力求车速/1 -> MinMax/2
  Constant9/1 -> Product3/1
  Add1/1 -> Product3/2
  Demux/3 -> MinMax/1
  Demux/1 -> Mux/1
  available drive force (N) brake force (N) and linear speed (m/s)/1 -> Demux/1
  Demux/2 -> 车轮制动力/1
  MinMax/1 -> Memory/1
  Memory/1 -> vehicle achievable consider of the road condition m/s/1

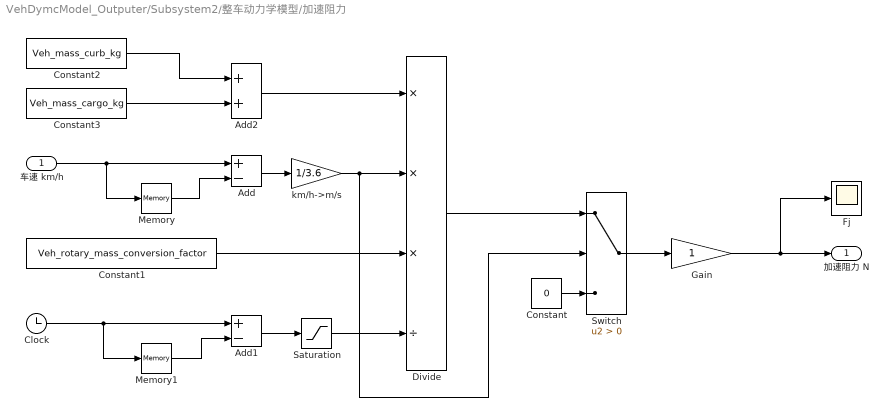
== system VehDymcModel_Outputer/Subsystem2/整车动力学模型/加速阻力 ==
  车速 km/h : Inport
  Add : Sum  Inputs=+-
  Add1 : Sum  Inputs=+-
  Add2 : Sum
  Clock : Clock
  Constant : Constant  Value=0
  Constant1 : Constant  Value=Veh_rotary_mass_conversion_factor
  Constant2 : Constant  Value=Veh_mass_curb_kg
  Constant3 : Constant  Value=Veh_mass_cargo_kg
  Divide : Product  Inputs=***/
  Fj : Scope
  Gain : Gain
  Memory : Memory  InheritSampleTime=on
  Memory1 : Memory
  Saturation : Saturate  UpperLimit=1.1  LowerLimit=0.9
  Switch : Switch  Criteria=u2 > Threshold  SaturateOnIntegerOverflow=off  InputSameDT=off
  km/h->m/s : Gain  Gain=1/3.6
  加速阻力 N : Outport
  wires:
  车速 km/h/1 -> Memory/1, Add/1
  Add/1 -> km/h->m/s/1
  km/h->m/s/1 -> Switch/2, Divide/2
  Gain/1 -> 加速阻力 N/1, Fj/1
  Memory/1 -> Add/2
  Memory1/1 -> Add1/2
  Add2/1 -> Divide/1
  Constant2/1 -> Add2/1
  Constant3/1 -> Add2/2
  Constant1/1 -> Divide/3
  Clock/1 -> Memory1/1, Add1/1
  Divide/1 -> Switch/1
  Constant/1 -> Switch/3
  Switch/1 -> Gain/1
  Add1/1 -> Saturation/1
  Saturation/1 -> Divide/4

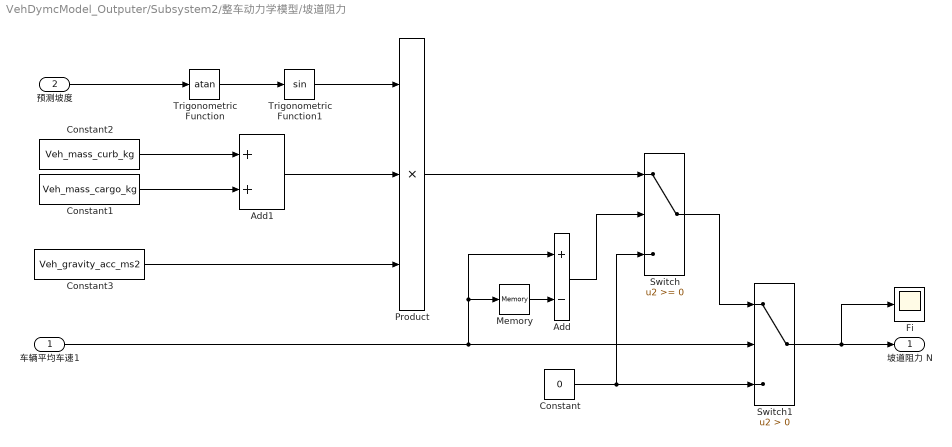
== system VehDymcModel_Outputer/Subsystem2/整车动力学模型/坡道阻力 ==
  车辆平均车速1 : Inport
  预测坡度 : Inport  Port=2
  Add : Sum  Inputs=+-
  Add1 : Sum
  Constant : Constant  Value=0
  Constant1 : Constant  Value=Veh_mass_cargo_kg
  Constant2 : Constant  Value=Veh_mass_curb_kg
  Constant3 : Constant  Value=Veh_gravity_acc_ms2
  Fi : Scope
  Memory : Memory  InheritSampleTime=on
  Product : Product  Inputs=3  RndMeth=Zero
  Switch : Switch  SaturateOnIntegerOverflow=off  InputSameDT=off
  Switch1 : Switch  Criteria=u2 > Threshold  SaturateOnIntegerOverflow=off  InputSameDT=off
  Trigonometric Function : Trigonometry  Operator=atan
  Trigonometric Function1 : Trigonometry
  坡道阻力 N : Outport
  wires:
  Trigonometric Function/1 -> Trigonometric Function1/1
  Trigonometric Function1/1 -> Product/1
  Constant3/1 -> Product/3
  Constant/1 -> Switch/3, Switch1/3
  预测坡度/1 -> Trigonometric Function/1
  Switch1/1 -> 坡道阻力 N/1, Fi/1
  Add1/1 -> Product/2
  Constant2/1 -> Add1/1
  Constant1/1 -> Add1/2
  车辆平均车速1/1 -> Add/1, Memory/1, Switch1/2
  Memory/1 -> Add/2
  Product/1 -> Switch/1
  Add/1 -> Switch/2
  Switch/1 -> Switch1/1

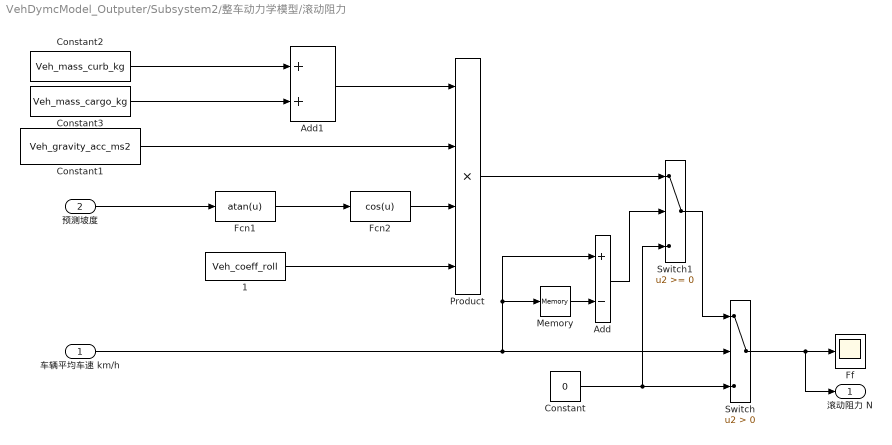
== system VehDymcModel_Outputer/Subsystem2/整车动力学模型/滚动阻力 ==
  车辆平均车速 km/h : Inport
  预测坡度 : Inport  Port=2
  "  1" : Constant  Value=Veh_coeff_roll
  Add : Sum  Inputs=+-
  Add1 : Sum
  Constant : Constant  Value=0
  Constant1 : Constant  Value=Veh_gravity_acc_ms2
  Constant2 : Constant  Value=Veh_mass_curb_kg
  Constant3 : Constant  Value=Veh_mass_cargo_kg
  Fcn1 : Fcn  Expr=atan(u)
  Fcn2 : Fcn  Expr=cos(u)
  Ff : Scope
  Memory : Memory  InheritSampleTime=on
  Product : Product  Inputs=4  RndMeth=Zero
  Switch : Switch  Criteria=u2 > Threshold  SaturateOnIntegerOverflow=off  InputSameDT=off
  Switch1 : Switch  SaturateOnIntegerOverflow=off  InputSameDT=off
  滚动阻力 N : Outport
  wires:
  Fcn2/1 -> Product/3
  Constant/1 -> Switch1/3, Switch/3
  Add1/1 -> Product/1
  Fcn1/1 -> Fcn2/1
  预测坡度/1 -> Fcn1/1
  Constant2/1 -> Add1/1
  Constant3/1 -> Add1/2
  车辆平均车速 km/h/1 -> Switch/2, Memory/1, Add/1
  Switch/1 -> Ff/1, 滚动阻力 N/1
  Constant1/1 -> Product/2
  "  1"/1 -> Product/4
  Product/1 -> Switch1/1
  Memory/1 -> Add/2
  Add/1 -> Switch1/2
  Switch1/1 -> Switch/1

== system VehDymcModel_Outputer/Subsystem2/整车动力学模型/空气阻力 ==
  veh_spd km/h : Inport
  Add : Sum  Inputs=-+
  Constant : Constant  Value=0
  Constant1 : Constant  Value=Veh_frontal_area_m2
  Constant2 : Constant  Value=Veh_coeff_drag
  Fw : Scope
  Gain : Gain  Gain=1/21.15
  Memory : Memory  InheritSampleTime=on
  Product : Product  Inputs=4  RndMeth=Zero
  Switch : Switch  SaturateOnIntegerOverflow=off  InputSameDT=off
  空气阻力 N : Outport
  wires:
  Constant1/1 -> Product/1
  Constant2/1 -> Product/2
  veh_spd km/h/1 -> Product/3, Memory/1, Add/2, Product/4
  Product/1 -> Gain/1
  Constant/1 -> Switch/3
  Gain/1 -> Switch/1
  Add/1 -> Switch/2
  Memory/1 -> Add/1
  Switch/1 -> Fw/1, 空气阻力 N/1

== system VehDymcModel_Outputer/Subsystem2/车轮模型/Interia torque ==
  note: This block computes the torque required to overcome the inertia of the
      | wheels and axle.
  车轮线速度 m/s : Inport
  Add : Sum  Inputs=+-
  Constant : Constant  Value=Veh_wheel_inertia
  Constant2 : Constant  Value=0
  Divide : Product  Inputs=**
  Memory : Memory  InheritSampleTime=on
  Switch : Switch  Criteria=u2 > Threshold  SaturateOnIntegerOverflow=off  InputSameDT=off
  axle input speed (rad/s) : Gain  Gain=1/Veh_wheel_radius_m
  inertia torque (Nm) : Outport  InitialOutput=0
  wires:
  Switch/1 -> Divide/1
  Constant/1 -> Divide/2
  Memory/1 -> Add/2
  axle input speed (rad/s)/1 -> Memory/1, Add/1
  车轮线速度 m/s/1 -> axle input speed (rad/s)/1
  Divide/1 -> inertia torque (Nm)/1
  Add/1 -> Switch/1, Switch/2
  Constant2/1 -> Switch/3

== system VehDymcModel_Outputer/Subsystem2/车轮模型/Interia torque1 ==
  note: This block computes the torque required to overcome the inertia of the
      | wheels and axle.
  车轮线速度 m/s : Inport
  Add : Sum  Inputs=+-
  Add1 : Sum  Inputs=+-
  Clock : Clock
  Constant : Constant  Value=Veh_wheel_inertia
  Constant2 : Constant  Value=0
  Divide : Product  Inputs=**/
  Memory : Memory  InheritSampleTime=on
  Memory1 : Memory  InheritSampleTime=on
  Saturation : Saturate  UpperLimit=1.1  LowerLimit=0.9
  Switch : Switch  SaturateOnIntegerOverflow=off  InputSameDT=off
  axle input speed (rad/s) : Gain  Gain=1/Veh_wheel_radius_m
  inertia torque (Nm) : Outport  InitialOutput=0
  wires:
  Switch/1 -> Divide/1
  Add/1 -> Switch/2, Switch/3
  Constant/1 -> Divide/2
  Memory1/1 -> Add1/2
  Clock/1 -> Memory1/1, Add1/1
  Memory/1 -> Add/2
  axle input speed (rad/s)/1 -> Memory/1, Add/1
  Constant2/1 -> Switch/1
  Add1/1 -> Saturation/1
  Saturation/1 -> Divide/3
  车轮线速度 m/s/1 -> axle input speed (rad/s)/1
  Divide/1 -> inertia torque (Nm)/1

== system VehDymcModel_Outputer/Subsystem2/车轮模型/Tire slip model ==
  In1 : Inport
  Add : Sum
  Constant : Constant  Value=Veh_gravity_acc_ms2
  Constant1 : Constant  Value=Veh_mass_curb_kg
  Constant2 : Constant  Value=Veh_mass_cargo_kg
  Constant3 : Constant  Value=Veh_wt_frac_front
  Constant4 : Constant  Value=Road_u
  Memory : Memory  InheritSampleTime=on
  MinMax : MinMax  Inputs=2  SampleTime=0
  Product : Product  Inputs=4  RndMeth=Zero
  dri_force available in front wheel n : Outport
  wires:
  Constant1/1 -> Add/1
  Constant2/1 -> Add/2
  Add/1 -> Product/3
  Constant3/1 -> Product/2
  Constant/1 -> Product/1
  Constant4/1 -> Product/4
  Product/1 -> Memory/1
  In1/1 -> MinMax/1
  MinMax/1 -> dri_force available in front wheel n/1
  Memory/1 -> MinMax/2

== system VehDymcModel_Outputer/Subsystem2/车轮模型/Tire slip model1 ==
  In1 : Inport
  Add : Sum
  Constant : Constant  Value=Veh_gravity_acc_ms2
  Constant1 : Constant  Value=Veh_mass_curb_kg
  Constant2 : Constant  Value=Veh_mass_cargo_kg
  Constant3 : Constant  Value=Veh_wt_frac_front
  Constant4 : Constant  Value=Road_u
  Gain1 : Gain  Gain=-1
  Memory : Memory  InheritSampleTime=on
  MinMax : MinMax  Function=max  Inputs=2  SampleTime=0
  Product : Product  Inputs=4  RndMeth=Zero
  brk_force available in front wheel n : Outport
  wires:
  Constant1/1 -> Add/1
  Constant2/1 -> Add/2
  Add/1 -> Product/3
  Constant3/1 -> Product/2
  Constant/1 -> Product/1
  Constant4/1 -> Product/4
  In1/1 -> MinMax/1
  MinMax/1 -> brk_force available in front wheel n/1
  Memory/1 -> MinMax/2
  Product/1 -> Gain1/1
  Gain1/1 -> Memory/1

== system VehDymcModel_Outputer/Subsystem2/驱动电机模型/Brake torque_limited ==
  tor_req nm : Inport
  mc spd rpm : Inport  Port=2
  1-D Lookup Table : Lookup_n-D  NumberOfTableDimensions=1  BreakpointsForDimension1=MC_ori_spd_rpm  Table=MC_ori_trq_brk_max_Nm  RndMeth=Simplest
  MinMax : MinMax  Function=max  Inputs=2
  limted mc torque nm : Outport
  wires:
  tor_req nm/1 -> MinMax/1
  mc spd rpm/1 -> 1-D Lookup Table/1
  1-D Lookup Table/1 -> MinMax/2
  MinMax/1 -> limted mc torque nm/1

== system VehDymcModel_Outputer/Subsystem2/驱动电机模型/Drive torque_limited ==
  tor_req nm : Inport
  mc spd rpm : Inport  Port=2
  1-D Lookup Table : Lookup_n-D  NumberOfTableDimensions=1  BreakpointsForDimension1=MC_ori_spd_rpm  Table=MC_ori_trq_dri_max_Nm  RndMeth=Simplest
  MinMax : MinMax  Inputs=2
  limted mc torque nm : Outport
  wires:
  tor_req nm/1 -> MinMax/1
  mc spd rpm/1 -> 1-D Lookup Table/1
  1-D Lookup Table/1 -> MinMax/2
  MinMax/1 -> limted mc torque nm/1

== system VehDymcModel_Outputer/Subsystem2/驱动电机模型/Inertia torque ==
  motor spd rpm : Inport
  Derivative : Derivative
  Gain1 : Gain  Gain=MC_inertia
  rpm->rad/s : Gain  Gain=2*pi/60
  Out1 : Outport
  wires:
  Derivative/1 -> Gain1/1
  Gain1/1 -> Out1/1
  rpm->rad/s/1 -> Derivative/1
  motor spd rpm/1 -> rpm->rad/s/1

== system VehDymcModel_Outputer/Subsystem2/驱动电机模型/Inertia torque1 ==
  motor spd rpm : Inport
  Derivative : Derivative
  Gain1 : Gain  Gain=MC_inertia
  rpm->rad/s : Gain  Gain=2*pi/60
  Out1 : Outport
  wires:
  Derivative/1 -> Gain1/1
  Gain1/1 -> Out1/1
  rpm->rad/s/1 -> Derivative/1
  motor spd rpm/1 -> rpm->rad/s/1

== system VehDymcModel_Outputer/Subsystem2/驱动电机模型/nm tor per pwr w input ==
  dri nm : Inport
  pwr dri kW : Inport  Port=2
  Add4 : Sum
  Constant : Constant  Value=eps
  Constant1 : Constant  Value=0
  Constant2 : Constant  Value=inf
  Divide : Product  Inputs=*/
  Relational Operator : RelationalOperator  Operator=~=  OutDataTypeStr=boolean  InputSameDT=off
  Switch : Switch  Threshold=eps  SaturateOnIntegerOverflow=off  InputSameDT=off
  kW->W : Gain  Gain=1000
  tor per pwr : Outport
  wires:
  Constant/1 -> Add4/2
  Add4/1 -> Divide/2
  dri nm/1 -> Divide/1
  Divide/1 -> Switch/1
  Constant1/1 -> Relational Operator/2
  Relational Operator/1 -> Switch/2
  Constant2/1 -> Switch/3
  pwr dri kW/1 -> kW->W/1
  Switch/1 -> tor per pwr/1
  kW->W/1 -> Add4/1, Relational Operator/1

== system VehDymcModel_Outputer/Subsystem2/驱动电机模型/nm tor per pwr w input1 ==
  pwr brk kW : Inport
  brk nm : Inport  Port=2
  Add4 : Sum
  Constant : Constant  Value=eps
  Constant1 : Constant  Value=0
  Constant2 : Constant  Value=inf
  Divide : Product  Inputs=*/
  Gain1 : Gain  Gain=-1
  Gain2 : Gain  Gain=-1000
  Relational Operator : RelationalOperator  Operator=~=  OutDataTypeStr=boolean  InputSameDT=off
  Switch : Switch  Threshold=eps  SaturateOnIntegerOverflow=off  InputSameDT=off
  tor per pwr : Outport
  wires:
  Gain2/1 -> Relational Operator/1, Add4/1
  Switch/1 -> tor per pwr/1
  Constant2/1 -> Switch/3
  Relational Operator/1 -> Switch/2
  Constant1/1 -> Relational Operator/2
  Divide/1 -> Switch/1
  Gain1/1 -> Divide/1
  Add4/1 -> Divide/2
  Constant/1 -> Add4/2
  pwr brk kW/1 -> Gain2/1
  brk nm/1 -> Gain1/1

== system VehDymcModel_Outputer/Subsystem2/驱动电机模型/rotor available brake torque nm ==
  tor per pwr : Inport
  pwr available kW : Inport  Port=2
  Constant : Constant  Value=inf
  Constant1 : Constant  Value=0
  Product : Product  RndMeth=Zero
  Relational Operator : RelationalOperator  Operator=~=  OutDataTypeStr=boolean  InputSameDT=off
  Switch : Switch  Threshold=0.3  SaturateOnIntegerOverflow=off  InputSameDT=off
  kW->W : Gain  Gain=1000
  tor avaible nm : Outport
  wires:
  Switch/1 -> tor avaible nm/1
  Constant1/1 -> Switch/3
  Relational Operator/1 -> Switch/2
  Constant/1 -> Relational Operator/2
  Product/1 -> Switch/1
  tor per pwr/1 -> Product/1, Relational Operator/1
  kW->W/1 -> Product/2
  pwr available kW/1 -> kW->W/1

== system VehDymcModel_Outputer/Subsystem2/驱动电机模型/rotor available drive torque nm ==
  tor per pwr : Inport
  pwr available kW : Inport  Port=2
  Constant : Constant  Value=inf
  Constant1 : Constant  Value=0
  Product : Product  RndMeth=Zero
  Relational Operator : RelationalOperator  Operator=~=  OutDataTypeStr=boolean  InputSameDT=off
  Switch : Switch  Threshold=0.3  SaturateOnIntegerOverflow=off  InputSameDT=off
  kW->W : Gain  Gain=1000
  tor avaible nm : Outport
  wires:
  Product/1 -> Switch/1
  Constant/1 -> Relational Operator/2
  Relational Operator/1 -> Switch/2
  Constant1/1 -> Switch/3
  tor per pwr/1 -> Product/1, Relational Operator/1
  Switch/1 -> tor avaible nm/1
  kW->W/1 -> Product/2
  pwr available kW/1 -> kW->W/1
